simulink model "GATING_SIGNALS01"  (R2022b)
settings: Solver=FixedStepAuto  StartTime=0.0  StopTime=10.0  RelTol=1e-3
model workspace (MAT data in the model file):
  g = 0.25
libraries: simulink x12, spsTriangleGeneratorLib x2
settings Model: Creator=amanp  LastModifiedBy=amanp
settings RTWCC: GenCodeOnly=on

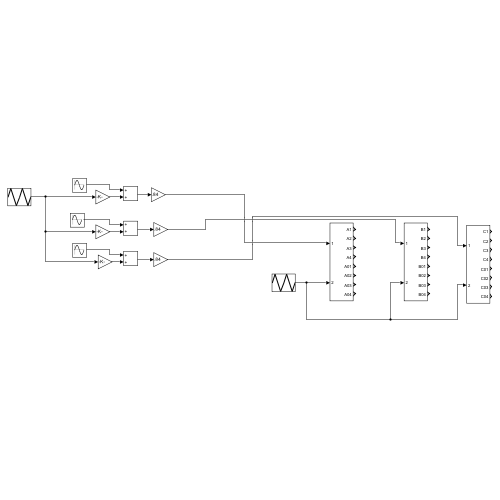
[thumbnail: Simulink's stored preview of the top-level diagram]
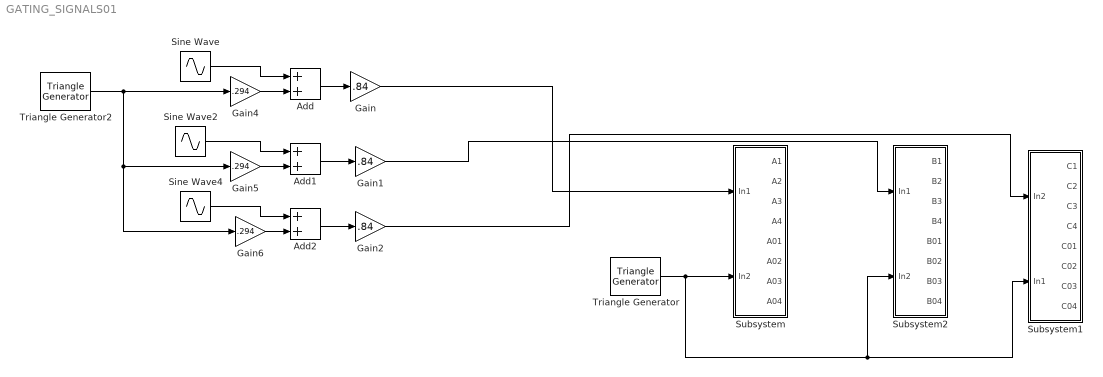
== system GATING_SIGNALS01 ==
  Add : Sum
  Add1 : Sum
  Add2 : Sum
  Gain : Gain  Gain=.84
  Gain1 : Gain  Gain=.84
  Gain2 : Gain  Gain=.84
  Gain4 : Gain  Gain=.294
  Gain5 : Gain  Gain=.294
  Gain6 : Gain  Gain=.294
  Sine Wave : Sin  Amplitude=1.92  Frequency=2*50*pi  SampleTime=0
  Sine Wave2 : Sin  Amplitude=1.92  Frequency=2*50*pi  Phase=2*pi/3  SampleTime=0
  Sine Wave4 : Sin  Amplitude=1.92  Frequency=2*50*pi  Phase=-2*pi/3  SampleTime=0
  Subsystem : Subsystem
  Subsystem1 : Subsystem
  Subsystem2 : Subsystem
  Triangle Generator : spsTriangleGeneratorLib/Triangle Generator  Freq=1e3*10  Phase=90  Ts=0
  Triangle Generator2 : spsTriangleGeneratorLib/Triangle Generator  Freq=150  Phase=90  Ts=0
  wires:
  Gain6/1 -> Add2/2
  Triangle Generator2/1 -> Gain6/1, Gain5/1, Gain4/1
  Add/1 -> Gain/1
  Add1/1 -> Gain1/1
  Gain/1 -> Subsystem/1(In1)
  Triangle Generator/1 -> Subsystem2/2(In2), Subsystem1/2(In1), Subsystem/2(In2)
  Sine Wave2/1 -> Add1/1
  Add2/1 -> Gain2/1
  Sine Wave4/1 -> Add2/1
  Gain2/1 -> Subsystem1/1(In2)
  Gain4/1 -> Add/2
  Gain1/1 -> Subsystem2/1(In1)
  Sine Wave/1 -> Add/1
  Gain5/1 -> Add1/2

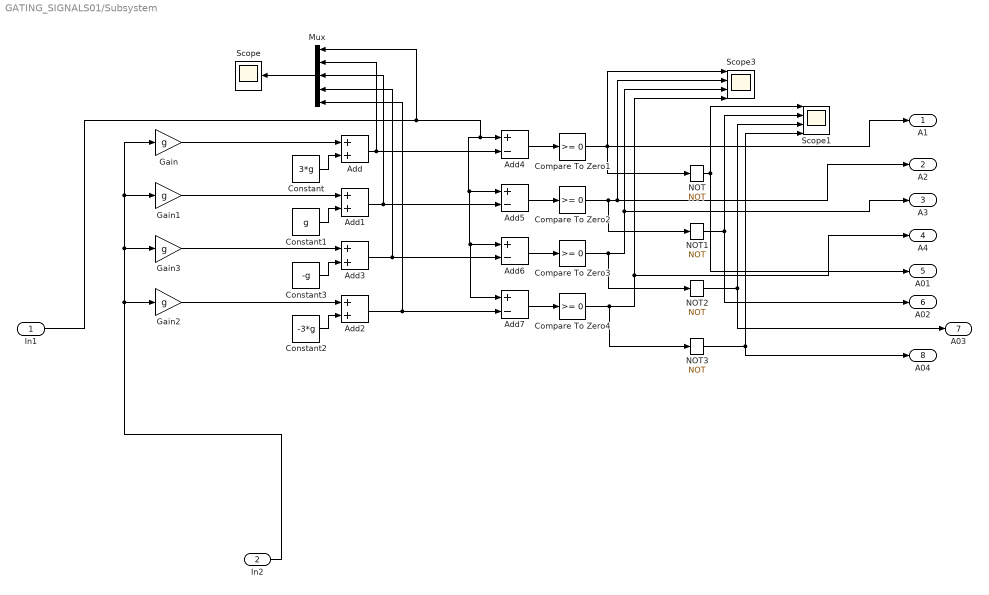
== system GATING_SIGNALS01/Subsystem ==
  In1 : Inport
  In2 : Inport  Port=2
  Add{,1..3} (4 alike) : Sum
  Add{4..7} (4 alike) : Sum  Inputs=+-
  Compare To Zero{1..4} (4 alike) : simulink/Logic and Bit Operations/Compare To Zero  relop=>=  OutDataTypeStr=boolean
  Constant : Constant  Value=3*g
  Constant1 : Constant  Value=g
  Constant2 : Constant  Value=-3*g
  Constant3 : Constant  Value=-g
  Gain{,1..3} (4 alike) : Gain  Gain=g
  Mux : Mux  Inputs=5
  NOT{,1..3} (4 alike) : Logic  Operator=NOT  IconShape=distinctive  AllPortsSameDT=off  OutDataTypeStr=boolean
  Scope : Scope
  Scope1 : Scope  NumInputPorts=4
  Scope3 : Scope  NumInputPorts=4
  A1 : Outport
  A2 : Outport  Port=2
  A3 : Outport  Port=3
  A4 : Outport  Port=4
  A01 : Outport  Port=5
  A02 : Outport  Port=6
  A03 : Outport  Port=7
  A04 : Outport  Port=8
  wires:
  Compare To Zero2/1 -> NOT1/1, A2/1, Scope3/2
  Add3/1 -> Mux/4, Add6/2
  Add/1 -> Mux/2, Add4/2
  Compare To Zero4/1 -> NOT3/1, Scope3/4, A4/1
  Add1/1 -> Mux/3, Add5/2
  In1/1 -> Mux/1, Add7/1, Add6/1, Add5/1, Add4/1
  Compare To Zero1/1 -> A1/1, Scope3/1, NOT/1
  In2/1 -> Gain1/1, Gain/1, Gain3/1, Gain2/1
  NOT1/1 -> A02/1, Scope1/2
  Gain1/1 -> Add1/1
  Gain/1 -> Add/1
  Constant/1 -> Add/2
  Add6/1 -> Compare To Zero3/1
  Add7/1 -> Compare To Zero4/1
  Constant3/1 -> Add3/2
  Add2/1 -> Mux/5, Add7/2
  Gain2/1 -> Add2/1
  Constant1/1 -> Add1/2
  Compare To Zero3/1 -> NOT2/1, A3/1, Scope3/3
  Constant2/1 -> Add2/2
  NOT/1 -> A01/1, Scope1/1
  Add5/1 -> Compare To Zero2/1
  Gain3/1 -> Add3/1
  Add4/1 -> Compare To Zero1/1
  NOT2/1 -> Scope1/3, A03/1
  NOT3/1 -> Scope1/4, A04/1
  Mux/1 -> Scope/1

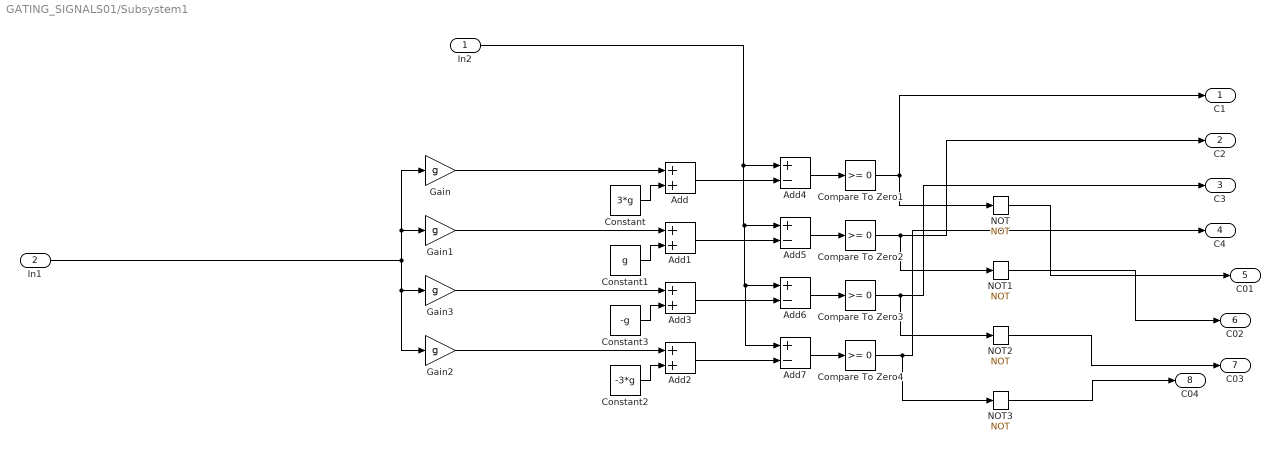
== system GATING_SIGNALS01/Subsystem1 ==
  In2 : Inport
  In1 : Inport  Port=2
  Add{,1..3} (4 alike) : Sum
  Add{4..7} (4 alike) : Sum  Inputs=+-
  Compare To Zero{1..4} (4 alike) : simulink/Logic and Bit Operations/Compare To Zero  relop=>=  OutDataTypeStr=boolean
  Constant : Constant  Value=3*g
  Constant1 : Constant  Value=g
  Constant2 : Constant  Value=-3*g
  Constant3 : Constant  Value=-g
  Gain{,1..3} (4 alike) : Gain  Gain=g
  NOT{,1..3} (4 alike) : Logic  Operator=NOT  IconShape=distinctive  AllPortsSameDT=off  OutDataTypeStr=boolean
  C1 : Outport
  C2 : Outport  Port=2
  C3 : Outport  Port=3
  C4 : Outport  Port=4
  C01 : Outport  Port=5
  C02 : Outport  Port=6
  C03 : Outport  Port=7
  C04 : Outport  Port=8
  wires:
  Add1/1 -> Add5/2
  In1/1 -> Gain1/1, Gain/1, Gain2/1, Gain3/1
  Gain1/1 -> Add1/1
  Compare To Zero1/1 -> C1/1, NOT/1
  Add7/1 -> Compare To Zero4/1
  Constant3/1 -> Add3/2
  Compare To Zero3/1 -> C3/1, NOT2/1
  Compare To Zero4/1 -> C4/1, NOT3/1
  Compare To Zero2/1 -> C2/1, NOT1/1
  Gain2/1 -> Add2/1
  Add5/1 -> Compare To Zero2/1
  Constant1/1 -> Add1/2
  In2/1 -> Add7/1, Add6/1, Add5/1, Add4/1
  Gain3/1 -> Add3/1
  Add6/1 -> Compare To Zero3/1
  Constant/1 -> Add/2
  NOT3/1 -> C04/1
  Add4/1 -> Compare To Zero1/1
  Constant2/1 -> Add2/2
  Add3/1 -> Add6/2
  Add/1 -> Add4/2
  NOT/1 -> C01/1
  Gain/1 -> Add/1
  Add2/1 -> Add7/2
  NOT1/1 -> C02/1
  NOT2/1 -> C03/1

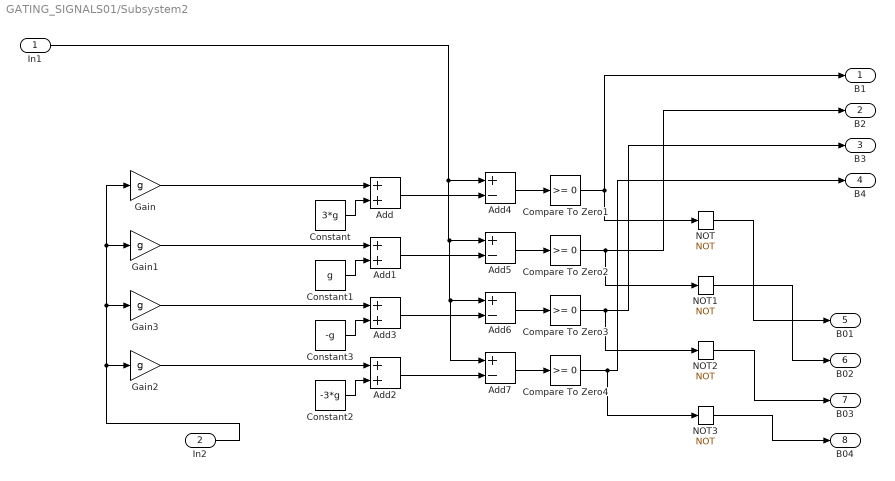
== system GATING_SIGNALS01/Subsystem2 ==
  In1 : Inport
  In2 : Inport  Port=2
  Add{,1..3} (4 alike) : Sum
  Add{4..7} (4 alike) : Sum  Inputs=+-
  Compare To Zero{1..4} (4 alike) : simulink/Logic and Bit Operations/Compare To Zero  relop=>=  OutDataTypeStr=boolean
  Constant : Constant  Value=3*g
  Constant1 : Constant  Value=g
  Constant2 : Constant  Value=-3*g
  Constant3 : Constant  Value=-g
  Gain{,1..3} (4 alike) : Gain  Gain=g
  NOT{,1..3} (4 alike) : Logic  Operator=NOT  IconShape=distinctive  AllPortsSameDT=off  OutDataTypeStr=boolean
  B1 : Outport
  B2 : Outport  Port=2
  B3 : Outport  Port=3
  B4 : Outport  Port=4
  B01 : Outport  Port=5
  B02 : Outport  Port=6
  B03 : Outport  Port=7
  B04 : Outport  Port=8
  wires:
  Constant/1 -> Add/2
  In2/1 -> Gain2/1, Gain3/1, Gain1/1, Gain/1
  Constant2/1 -> Add2/2
  Gain1/1 -> Add1/1
  Add2/1 -> Add7/2
  Compare To Zero3/1 -> B3/1, NOT2/1
  Add1/1 -> Add5/2
  NOT1/1 -> B02/1
  Compare To Zero2/1 -> B2/1, NOT1/1
  Compare To Zero1/1 -> B1/1, NOT/1
  Add4/1 -> Compare To Zero1/1
  Compare To Zero4/1 -> B4/1, NOT3/1
  Add3/1 -> Add6/2
  In1/1 -> Add4/1, Add5/1, Add6/1, Add7/1
  Add6/1 -> Compare To Zero3/1
  Add/1 -> Add4/2
  Add5/1 -> Compare To Zero2/1
  NOT2/1 -> B03/1
  Gain/1 -> Add/1
  Gain2/1 -> Add2/1
  Constant1/1 -> Add1/2
  Add7/1 -> Compare To Zero4/1
  Constant3/1 -> Add3/2
  NOT3/1 -> B04/1
  Gain3/1 -> Add3/1
  NOT/1 -> B01/1
